simulink model "LateralSim"  (Simulink 8.7)
settings: Solver=FixedStepDiscrete  StartTime=0.0  StopTime=100  FixedStep=0.002  RelTol=1e-3
undefined symbols (not defined in the file or in its folder): DiscIntNeverNeededParam
settings Model: Creator=cbeal  LastModifiedBy=cbeal
settings SolverCC: InitialStep=.001  ZeroCrossAlgorithm=Adaptive
settings DataIOCC: LimitDataPoints=off  SignalLoggingSaveFormat=ModelDataLogs  Refine=5
settings OptimizationCC: ExpressionDepthLimit=2147483647
settings DebuggingCC: SolverPrmCheckMsg=warning  FcnCallInpInsideContextMsg=EnableAllAsWarning  StateNameClashWarn=warning
settings ConfigComp: CovSFcnEnable=off

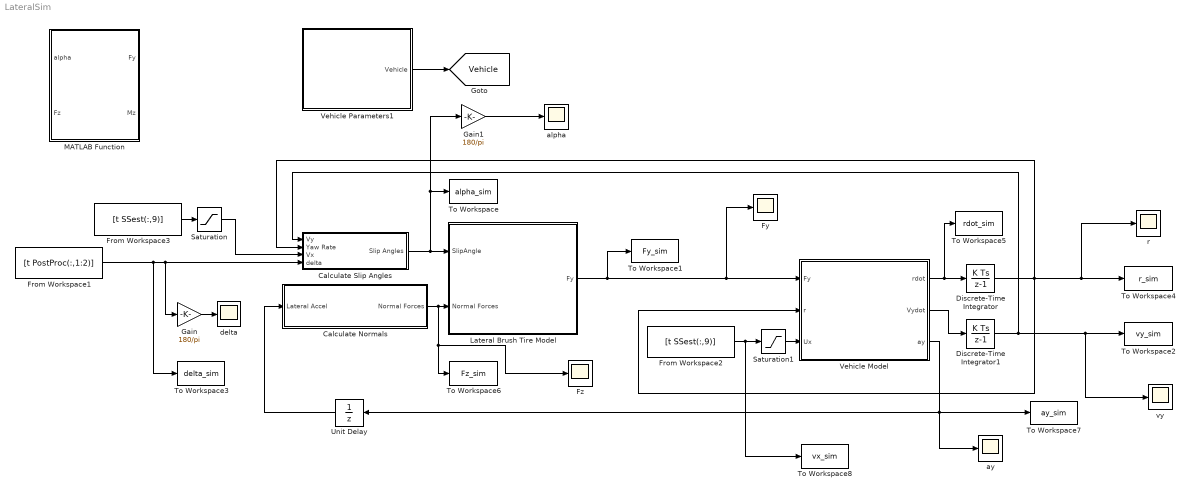
== system LateralSim ==
  Calculate Normals : Subsystem
  Calculate Slip Angles : Subsystem
  Discrete-Time Integrator : DiscreteIntegrator  InitialConditionSetting=State (most efficient)  SampleTime=-1  ICPrevOutput=DiscIntNeverNeededParam  ICPrevScaledInput=DiscIntNeverNeededParam
  Discrete-Time Integrator1 : DiscreteIntegrator  InitialConditionSetting=State (most efficient)  SampleTime=-1  ICPrevOutput=DiscIntNeverNeededParam  ICPrevScaledInput=DiscIntNeverNeededParam
  From Workspace1 : FromWorkspace  VariableName=[t PostProc(:,1:2)]  SampleTime=0  OutputAfterFinalValue=Setting to zero
  From Workspace2 : FromWorkspace  VariableName=[t SSest(:,9)]  SampleTime=0  OutputAfterFinalValue=Setting to zero
  From Workspace3 : FromWorkspace  VariableName=[t SSest(:,9)]  SampleTime=0  OutputAfterFinalValue=Setting to zero
  Fy : Scope
  Fz : Scope
  Gain : Gain  Gain=180/pi
  Gain1 : Gain  Gain=180/pi
  Lateral Brush Tire Model : Subsystem
  MATLAB Function : MATLAB Function  TreatAsAtomicUnit=on  mask{Ca=50000*ones(4,1), mu=[1.4; 1.4; 1.0; 1.0], muRatio=1*ones(4,1), CaShapeA=2.43*ones(4,1), CaShapeB=1.54*ones(4,1), aShape=0.278*ones(4,1)}
      mask prompts: Ca "Cornering Stiffness"; mu "Adhesion Friction"; muRatio "Sliding/Adhesion Ratio"; CaShapeA "Cornering Stiffness Shape Factor A"; CaShapeB "Cornering Stiffness Shape Factor B"; aShape "Contact Patch Length Factor"
  Saturation : Saturate  UpperLimit=inf  LowerLimit=0.3
  Saturation1 : Saturate  UpperLimit=inf  LowerLimit=0.3
  To Workspace : ToWorkspace  VariableName=alpha_sim  SampleTime=-1
  To Workspace1 : ToWorkspace  VariableName=Fy_sim  SampleTime=-1
  To Workspace2 : ToWorkspace  VariableName=vy_sim  SampleTime=-1
  To Workspace3 : ToWorkspace  VariableName=delta_sim  SampleTime=-1
  To Workspace4 : ToWorkspace  VariableName=r_sim  SampleTime=-1
  To Workspace5 : ToWorkspace  VariableName=rdot_sim  SampleTime=-1
  To Workspace6 : ToWorkspace  VariableName=Fz_sim  SampleTime=-1
  To Workspace7 : ToWorkspace  VariableName=ay_sim  SampleTime=-1
  To Workspace8 : ToWorkspace  VariableName=vx_sim  SampleTime=-1
  Unit Delay : UnitDelay  SampleTime=-1
  Vehicle Model : Subsystem
  Vehicle Parameters1 : Subsystem  mask{vehicleName='P1', m=1725, m_s=1680, Ixx=0, Iyy=0, Izz=1150, Iw=1.2, Re=0.32, a=1.35, b=1.15, d=1.63, h_cg=0.35, h_rcf=0, h_rcr=0, k_phi=[80000,80000], b_phi=[2400, 2400], Ca=[45000; 45000; 62000; 62000], Cx=[30000; 30000; 30000; 30000], mu_peak=[1.6 1.6 1.2 1.2], mu_slide=[1.4 1.4 0.9 0.9]}
      mask prompts: vehicleName "Name of Vehicle"; m "Mass"; m_s "Sprung Mass"; Ixx "Roll Moment of Inertia"; Iyy "Pitch Moment of Inertia"; Izz "Yaw Moment of Inertia"; Iw "Wheel Moment of Inertia"; Re "Wheel Effective Radius"; a "CG-Front Axle Distance"; b "CG-Rear Axle Distance"; d "Track Width"; h_cg "CG height"; h_rcf "Front Roll Center Height"; h_rcr "Rear Roll Center Height"; k_phi "Chassis Roll Stiffness (x2)"; b_phi "Chassis Roll Damping (x2)"; Ca "Cornering Stiffnesses (x4)"; Cx "Longitudinal Stiffnesses (x4)"; mu_peak "Peak Coeff. Friction (x4)"; mu_slide "Sliding Coeff. Friction (x4)"
      mask Display: port_label('output',1,vehicleName)
  alpha : Scope
  ay : Scope
  delta : Scope
  r : Scope
  vy : Scope
  tag scope: Vehicle=global
  wires:
  Calculate Slip Angles/1(Slip Angles) -> Lateral Brush Tire Model/1(SlipAngle), To Workspace/1, Gain1/1
  Vehicle Model/1(rdot) -> Discrete-Time Integrator/1, To Workspace5/1
  Discrete-Time Integrator/1 -> Calculate Slip Angles/2(Yaw Rate), Vehicle Model/2(r), To Workspace4/1, r/1
  Discrete-Time Integrator1/1 -> Calculate Slip Angles/1(Vy), To Workspace2/1, vy/1
  Lateral Brush Tire Model/1(Fy) -> To Workspace1/1, Vehicle Model/1(Fy), Fy/1
  Calculate Normals/1(Normal Forces) -> Lateral Brush Tire Model/2(Normal Forces), To Workspace6/1, Fz/1
  Vehicle Model/2(Vydot) -> Discrete-Time Integrator1/1
  Vehicle Model/3(ay) -> Unit Delay/1, To Workspace7/1, ay/1
  From Workspace3/1 -> Saturation/1
  From Workspace2/1 -> To Workspace8/1, Saturation1/1
  Gain/1 -> delta/1
  Gain1/1 -> alpha/1
  Vehicle Parameters1/1(Vehicle) -> [Vehicle]
  From Workspace1/1 -> Calculate Slip Angles/4(delta), Gain/1, To Workspace3/1
  Saturation/1 -> Calculate Slip Angles/3(Vx)
  Saturation1/1 -> Vehicle Model/3(Ux)
  Unit Delay/1 -> Calculate Normals/1(Lateral Accel)

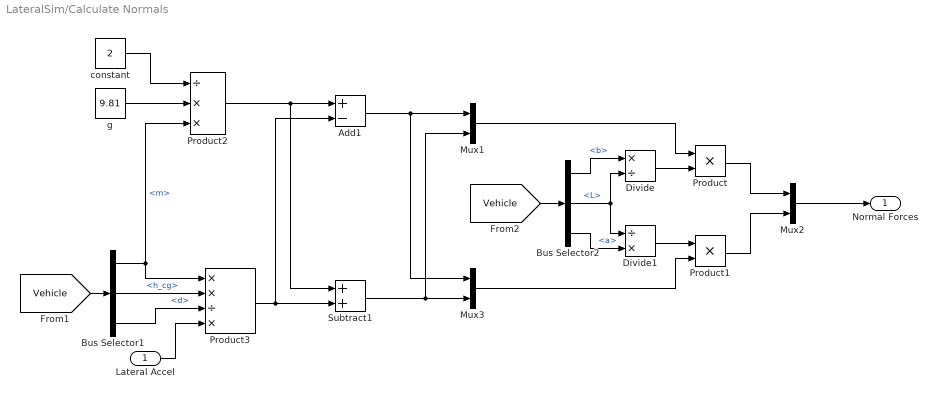
== system LateralSim/Calculate Normals ==
  Lateral Accel : Inport
  Add1 : Sum  Inputs=+-
  Bus Selector1 : BusSelector  OutputSignals=m,h_cg,d
  Bus Selector2 : BusSelector  OutputSignals=b,L,a
  Divide : Product  Inputs=*/
  Divide1 : Product  Inputs=/*
  Mux1 : Mux  Inputs=2
  Mux2 : Mux  Inputs=2
  Mux3 : Mux  Inputs=2
  Product : Product  RndMeth=Zero
  Product1 : Product  RndMeth=Zero
  Product2 : Product  Inputs=/**  RndMeth=Zero
  Product3 : Product  Inputs=**/*  RndMeth=Zero
  Subtract1 : Sum
  constant : Constant  Value=2
  g : Constant  Value=9.81
  Normal Forces : Outport
  wires:
  [Vehicle] -> Bus Selector1/1
  Mux2/1 -> Normal Forces/1
  Bus Selector1/1 -> Product3/1, Product2/3  "<m>"
  Bus Selector1/2 -> Product3/2  "<h_cg>"
  Bus Selector1/3 -> Product3/3  "<d>"
  Lateral Accel/1 -> Product3/4
  Product3/1 -> Subtract1/2, Add1/2
  g/1 -> Product2/2
  constant/1 -> Product2/1
  Product2/1 -> Add1/1, Subtract1/1
  [Vehicle] -> Bus Selector2/1
  Bus Selector2/2 -> Divide/2, Divide1/1  "<L>"
  Divide1/1 -> Product1/1
  Divide/1 -> Product/2
  Bus Selector2/1 -> Divide/1  "<b>"
  Bus Selector2/3 -> Divide1/2  "<a>"
  Add1/1 -> Mux1/1, Mux3/1
  Subtract1/1 -> Mux3/2, Mux1/2
  Product1/1 -> Mux2/2
  Product/1 -> Mux2/1
  Mux1/1 -> Product/1
  Mux3/1 -> Product1/2

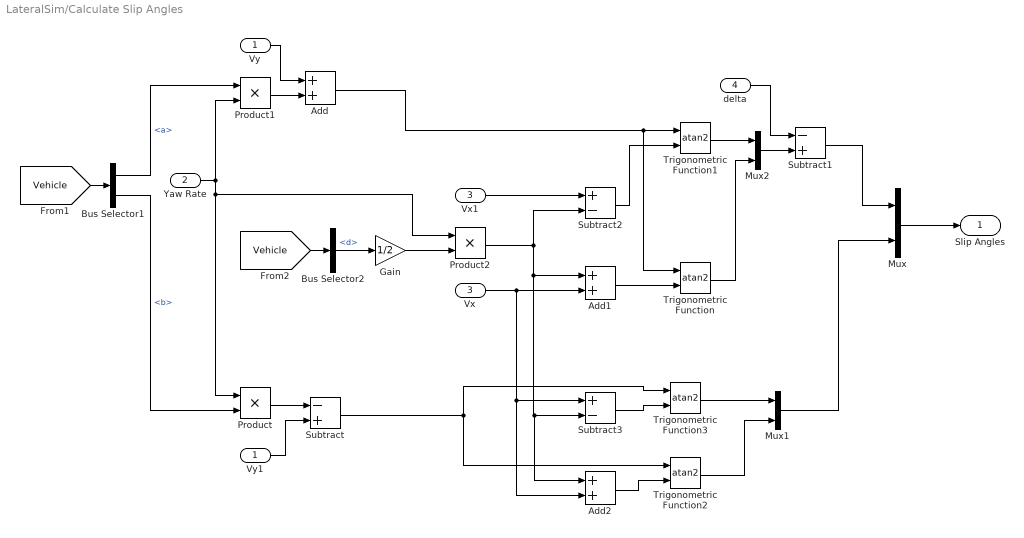
== system LateralSim/Calculate Slip Angles ==
  Vy : Inport
  Yaw Rate : Inport  Port=2
  Vx : Inport  Port=3
  delta : Inport  Port=4
  Add : Sum
  Add1 : Sum
  Add2 : Sum
  Bus Selector1 : BusSelector  OutputSignals=a,b
  Bus Selector2 : BusSelector  OutputSignals=d
  Gain : Gain  Gain=1/2
  Mux : Mux  Inputs=2
  Mux1 : Mux  Inputs=2
  Mux2 : Mux  Inputs=2
  Product : Product  RndMeth=Zero
  Product1 : Product  RndMeth=Zero
  Product2 : Product  RndMeth=Zero
  Subtract : Sum  Inputs=-+
  Subtract1 : Sum  Inputs=-+
  Subtract2 : Sum  Inputs=+-
  Subtract3 : Sum  Inputs=+-
  Trigonometric Function{,1..3} (4 alike) : Trigonometry  Operator=atan2
  Vx1 : InportShadow  Port=3
  Vy1 : InportShadow
  Slip Angles : Outport
  wires:
  [Vehicle] -> Bus Selector1/1
  Yaw Rate/1 -> Product2/1, Product/1, Product1/2
  Bus Selector1/1 -> Product1/1  "<a>"
  Bus Selector1/2 -> Product/2  "<b>"
  Product/1 -> Subtract/1
  Vy1/1 -> Subtract/2
  Mux/1 -> Slip Angles/1
  Product1/1 -> Add/2
  Add/1 -> Trigonometric Function1/1, Trigonometric Function/1
  Vy/1 -> Add/1
  Subtract1/1 -> Mux/1
  Mux1/1 -> Mux/2
  delta/1 -> Subtract1/1
  Mux2/1 -> Subtract1/2
  Trigonometric Function1/1 -> Mux2/1
  [Vehicle] -> Bus Selector2/1
  Bus Selector2/1 -> Gain/1  "<d>"
  Gain/1 -> Product2/2
  Vx1/1 -> Subtract2/1
  Product2/1 -> Add2/1, Subtract3/2, Add1/1, Subtract2/2
  Vx/1 -> Subtract3/1, Add2/2, Add1/2
  Trigonometric Function/1 -> Mux2/2
  Subtract2/1 -> Trigonometric Function1/2
  Add1/1 -> Trigonometric Function/2
  Trigonometric Function3/1 -> Mux1/1
  Trigonometric Function2/1 -> Mux1/2
  Subtract3/1 -> Trigonometric Function3/2
  Add2/1 -> Trigonometric Function2/2
  Subtract/1 -> Trigonometric Function2/1, Trigonometric Function3/1

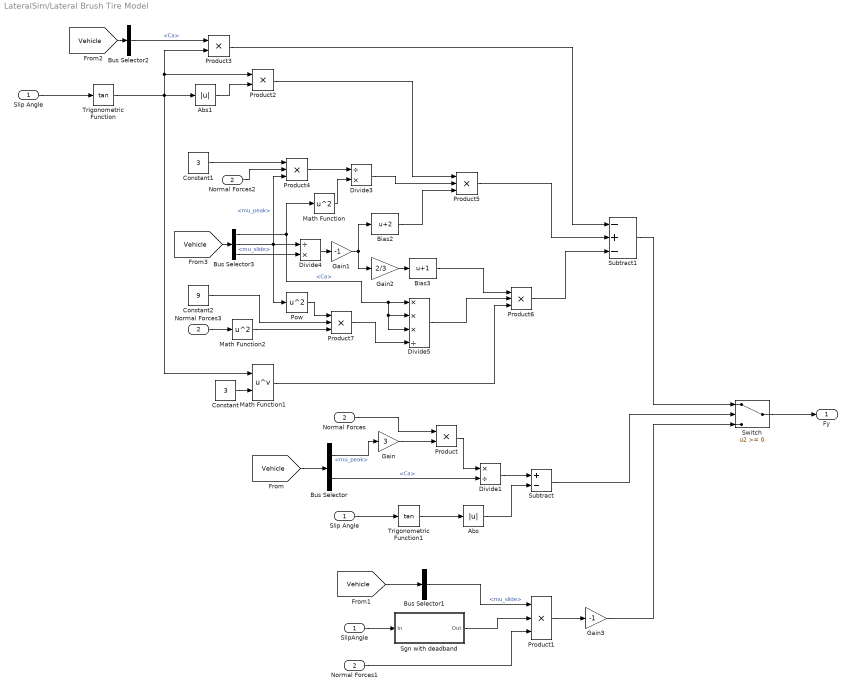
== system LateralSim/Lateral Brush Tire Model ==
  SlipAngle : Inport
  Normal Forces : Inport  Port=2
  Abs : Abs  ZeroCross=off
  Abs1 : Abs  ZeroCross=off
  Bias2 : Bias  Bias=2
  Bias3 : Bias  Bias=1
  Bus Selector : BusSelector  OutputSignals=mu_peak,Ca
  Bus Selector1 : BusSelector  OutputSignals=mu_slide
  Bus Selector2 : BusSelector  OutputSignals=Ca
  Bus Selector3 : BusSelector  OutputSignals=Ca,mu_peak,mu_slide
  Constant : Constant  Value=3
  Constant1 : Constant  Value=3
  Constant2 : Constant  Value=9
  Divide1 : Product  Inputs=*/
  Divide3 : Product  Inputs=/*
  Divide4 : Product  Inputs=/*
  Divide5 : Product  Inputs=***/
  Gain : Gain  Gain=3
  Gain1 : Gain  Gain=-1
  Gain2 : Gain  Gain=2/3
  Gain3 : Gain  Gain=-1
  Math Function : Math  Operator=square  SaturateOnIntegerOverflow=on
  Math Function1 : Math  Operator=pow  SaturateOnIntegerOverflow=on
  Math Function2 : Math  Operator=square  SaturateOnIntegerOverflow=on
  Normal Forces1 : InportShadow  Port=2
  Normal Forces2 : InportShadow  Port=2
  Normal Forces3 : InportShadow  Port=2
  Pow : Math  Operator=square  SaturateOnIntegerOverflow=on
  Product : Product  RndMeth=Zero
  Product{1,4..7} (5 alike) : Product  Inputs=3  RndMeth=Zero
  Product2 : Product  RndMeth=Zero
  Product3 : Product  RndMeth=Zero
  Sgn with deadband : Subsystem  mask{lower_dz=-0.01, upper_dz=0.01}
      mask prompts: lower_dz "Lower Dead Zone Boundary"; upper_dz "Upper Dead Zone Boundary"
  Slip Angle : InportShadow
  "Slip Angle " : InportShadow
  Subtract : Sum  Inputs=+-
  Subtract1 : Sum  Inputs=-+-
  Switch : Switch
  Trigonometric Function : Trigonometry  Operator=tan
  Trigonometric Function1 : Trigonometry  Operator=tan
  Fy : Outport
  wires:
  [Vehicle] -> Bus Selector/1
  Trigonometric Function1/1 -> Abs/1
  Abs/1 -> Subtract/2
  Bus Selector/2 -> Divide1/2  "<Ca>"
  Divide1/1 -> Subtract/1
  Normal Forces/1 -> Product/1
  Product/1 -> Divide1/1
  Bus Selector/1 -> Gain/1  "<mu_peak>"
  Gain/1 -> Product/2
  Switch/1 -> Fy/1
  SlipAngle/1 -> Sgn with deadband/1(In)
  [Vehicle] -> Bus Selector1/1
  Bus Selector1/1 -> Product1/1  "<mu_slide>"
  Sgn with deadband/1(Out) -> Product1/2
  Normal Forces1/1 -> Product1/3
  [Vehicle] -> Bus Selector2/1
  Trigonometric Function/1 -> Abs1/1, Math Function1/1, Product2/1, Product3/2
  Slip Angle/1 -> Trigonometric Function/1
  Constant/1 -> Math Function1/2
  Abs1/1 -> Product2/2
  Bus Selector2/1 -> Product3/1  "<Ca>"
  Product3/1 -> Subtract1/1
  [Vehicle] -> Bus Selector3/1
  Constant1/1 -> Product4/1
  Normal Forces2/1 -> Product4/2
  Bus Selector3/2 -> Divide4/1, Product4/3, Pow/1  "<mu_peak>"
  Bus Selector3/1 -> Math Function/1, Divide5/1, Divide5/2, Divide5/3  "<Ca>"
  Product4/1 -> Divide3/1
  Math Function/1 -> Divide3/2
  Bus Selector3/3 -> Divide4/2  "<mu_slide>"
  Divide4/1 -> Gain1/1
  Gain1/1 -> Bias2/1, Gain2/1
  Gain2/1 -> Bias3/1
  Bias2/1 -> Product5/3
  Divide3/1 -> Product5/2
  Product2/1 -> Product5/1
  Product5/1 -> Subtract1/2
  Math Function1/1 -> Product6/3
  Bias3/1 -> Product6/1
  Normal Forces3/1 -> Math Function2/1
  Constant2/1 -> Product7/2
  Math Function2/1 -> Product7/3
  Pow/1 -> Product7/1
  Divide5/1 -> Product6/2
  Product6/1 -> Subtract1/3
  Subtract1/1 -> Switch/1
  Product7/1 -> Divide5/4
  Product1/1 -> Gain3/1
  Subtract/1 -> Switch/2
  "Slip Angle "/1 -> Trigonometric Function1/1
  Gain3/1 -> Switch/3

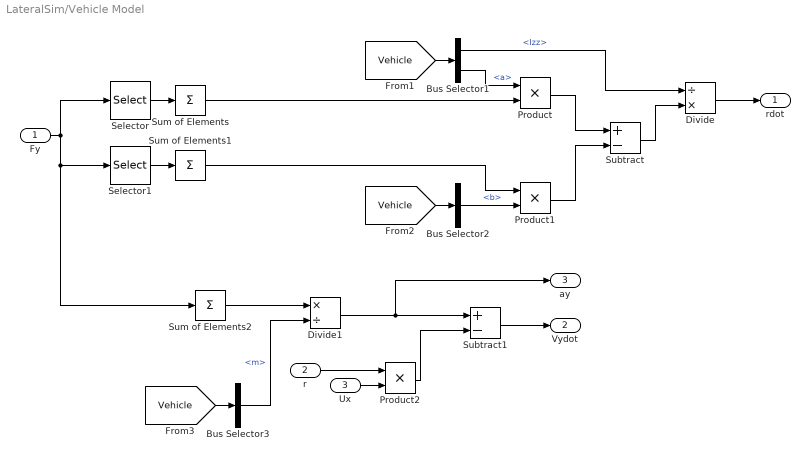
== system LateralSim/Vehicle Model ==
  Fy : Inport
  r : Inport  Port=2
  Ux : Inport  Port=3
  Bus Selector1 : BusSelector  OutputSignals=Izz,a
  Bus Selector2 : BusSelector  OutputSignals=b
  Bus Selector3 : BusSelector  OutputSignals=m
  Divide : Product  Inputs=/*
  Divide1 : Product  Inputs=*/
  Product : Product  RndMeth=Zero
  Product1 : Product  RndMeth=Zero
  Product2 : Product  RndMeth=Zero
  Selector : Selector  InputPortWidth=4  IndexOptions=Index vector (dialog)  Indices=[1 2]  OutputSizes=1
  Selector1 : Selector  InputPortWidth=4  IndexOptions=Index vector (dialog)  Indices=[3 4]  OutputSizes=1
  Subtract : Sum  Inputs=+-
  Subtract1 : Sum  Inputs=+-
  Sum of Elements : Sum  Inputs=+
  Sum of Elements1 : Sum  Inputs=+
  Sum of Elements2 : Sum  Inputs=+
  rdot : Outport
  Vydot : Outport  Port=2
  ay : Outport  Port=3
  wires:
  Fy/1 -> Selector/1, Selector1/1, Sum of Elements2/1
  Divide/1 -> rdot/1
  [Vehicle] -> Bus Selector1/1
  Selector/1 -> Sum of Elements/1
  Selector1/1 -> Sum of Elements1/1
  Sum of Elements/1 -> Product/2
  Bus Selector1/2 -> Product/1  "<a>"
  [Vehicle] -> Bus Selector2/1
  Sum of Elements1/1 -> Product1/1
  Bus Selector2/1 -> Product1/2  "<b>"
  Bus Selector1/1 -> Divide/1  "<Izz>"
  Product/1 -> Subtract/1
  Product1/1 -> Subtract/2
  Subtract/1 -> Divide/2
  [Vehicle] -> Bus Selector3/1
  Sum of Elements2/1 -> Divide1/1
  Bus Selector3/1 -> Divide1/2  "<m>"
  Divide1/1 -> Subtract1/1, ay/1
  Subtract1/1 -> Vydot/1
  Ux/1 -> Product2/2
  r/1 -> Product2/1
  Product2/1 -> Subtract1/2

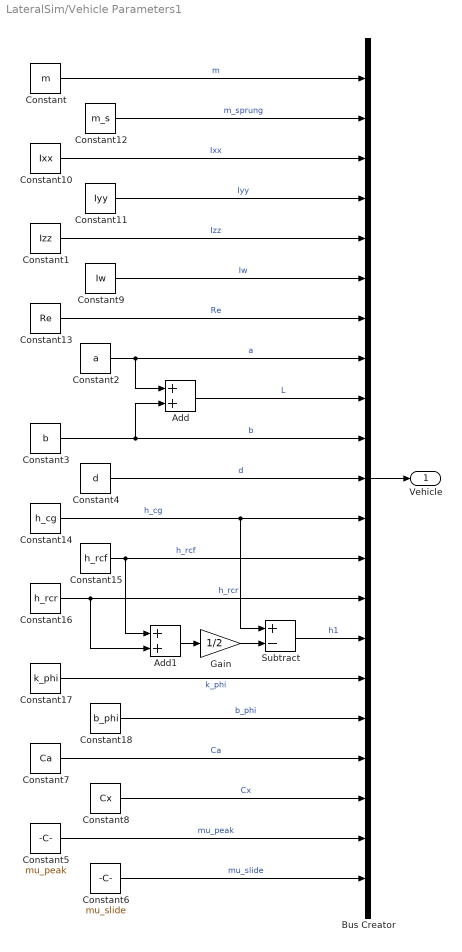
== system LateralSim/Vehicle Parameters1 ==
  Add : Sum
  Add1 : Sum
  Bus Creator : BusCreator  Inputs=21
  Constant : Constant  Value=m
  Constant1 : Constant  Value=Izz
  Constant10 : Constant  Value=Ixx
  Constant11 : Constant  Value=Iyy
  Constant12 : Constant  Value=m_s
  Constant13 : Constant  Value=Re
  Constant14 : Constant  Value=h_cg
  Constant15 : Constant  Value=h_rcf
  Constant16 : Constant  Value=h_rcr
  Constant17 : Constant  Value=k_phi
  Constant18 : Constant  Value=b_phi
  Constant2 : Constant  Value=a
  Constant3 : Constant  Value=b
  Constant4 : Constant  Value=d
  Constant5 : Constant  Value=mu_peak
  Constant6 : Constant  Value=mu_slide
  Constant7 : Constant  Value=Ca
  Constant8 : Constant  Value=Cx
  Constant9 : Constant  Value=Iw
  Gain : Gain  Gain=1/2
  Subtract : Sum  Inputs=+-
  Vehicle : Outport
  wires:
  Constant2/1 -> Add/1, Bus Creator/8  "a"
  Constant3/1 -> Add/2, Bus Creator/10  "b"
  Bus Creator/1 -> Vehicle/1
  Constant/1 -> Bus Creator/1  "m"
  Constant12/1 -> Bus Creator/2  "m_sprung"
  Constant10/1 -> Bus Creator/3  "Ixx"
  Constant11/1 -> Bus Creator/4  "Iyy"
  Constant1/1 -> Bus Creator/5  "Izz"
  Constant9/1 -> Bus Creator/6  "Iw"
  Constant13/1 -> Bus Creator/7  "Re"
  Add/1 -> Bus Creator/9  "L"
  Constant4/1 -> Bus Creator/11  "d"
  Constant14/1 -> Bus Creator/12, Subtract/1  "h_cg"
  Constant15/1 -> Bus Creator/13, Add1/1  "h_rcf"
  Constant16/1 -> Bus Creator/14, Add1/2  "h_rcr"
  Constant17/1 -> Bus Creator/16  "k_phi"
  Constant18/1 -> Bus Creator/17  "b_phi"
  Constant7/1 -> Bus Creator/18  "Ca"
  Constant8/1 -> Bus Creator/19  "Cx"
  Constant5/1 -> Bus Creator/20  "mu_peak"
  Constant6/1 -> Bus Creator/21  "mu_slide"
  Subtract/1 -> Bus Creator/15  "h1"
  Add1/1 -> Gain/1
  Gain/1 -> Subtract/2

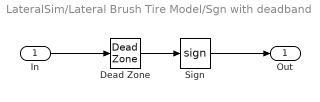
== system LateralSim/Lateral Brush Tire Model/Sgn with deadband ==
  In : Inport
  Dead Zone : DeadZone  LowerValue=-lower_dz  UpperValue=upper_dz  ZeroCross=off  SaturateOnIntegerOverflow=on
  Sign : Signum  ZeroCross=off
  Out : Outport
  wires:
  In/1 -> Dead Zone/1
  Dead Zone/1 -> Sign/1
  Sign/1 -> Out/1

== matlab function MATLAB Function ==
  data: alpha input double; Fy output double; Fz input double; mu parameter double; Ca parameter double; muRatio parameter double; CaShapeA parameter double; CaShapeB parameter double; aShape parameter double; Mz output double
function [Fy,Mz] = fcn(alpha,Fz,mu, Ca, muRatio, CaShapeA, CaShapeB, aShape)

Calpha = Ca.*sin(CaShapeA.*atan(CaShapeB*1e-4.*Fz));   % from Chris' notes (see adaption from Pacejka using variable a with c_{px} instead of C_\alpha)
mup = mu - (2e-5)*Fz;                    % from Chris' notes
mus = mu.*muRatio - (2e-5)*Fz;                  % from Chris' notes
sigmay = tan(alpha);
asq = aShape.*Fz*1.5e-4; % half contact patch length

if(any(asq < 0))
    disp('asq less than 0');
    Fz
end

% Compute the forces and moments
Fy = -Calpha.*sigmay + Calpha.^2./(3*mup.*Fz).*(2-mus./mup).*abs(sigmay).*sigmay - Calpha.^3./(9*(mup.*Fz).^2).*(1-2/3*mus./mup).*sigmay.^3;
Mz = sqrt(asq).*sigmay.*Calpha/3.*(1 - Calpha.*abs(sigmay)./(mup.*Fz).*(2-mus./mup) + (Calpha.*sigmay./(mup.*Fz)).^2.*(1-2/3*mus./mup) - (Calpha.*abs(sigmay)./(mup.*Fz)).^3.*(4/27 - 1/9*mus./mup));
satInds = abs(alpha) > 3*mup.*Fz./(Calpha);
Fy(satInds) = -sign(alpha(satInds)).*mus(satInds).*Fz(satInds);
Mz(satInds) = 0;
